simulink model "PhantomOmniSimulink"  (R2017b)
settings: Solver=VariableStepAuto  StartTime=0.0  StopTime=10.0  RelTol=1e-3
settings Model: Creator=nomad  LastModifiedBy=nomad

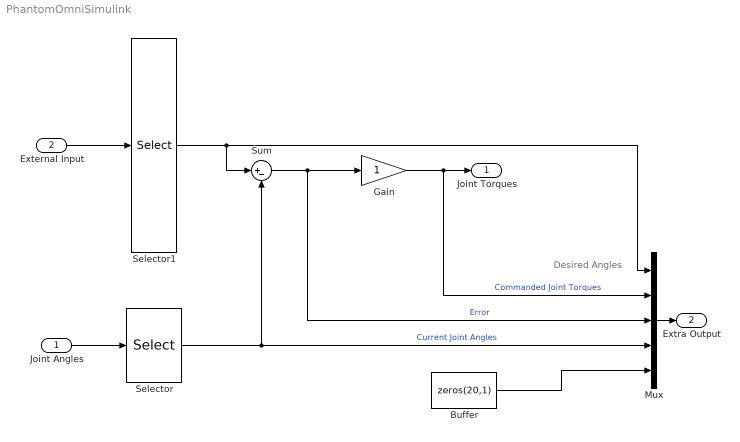
== system PhantomOmniSimulink ==
  note: Desired Angles
  Joint Angles : Inport  PortDimensions=6
  External Input : Inport  Port=2  PortDimensions=16
  Buffer : Constant  Value=zeros(20,1)
  Gain : Gain
  Mux : Mux  Inputs=5
  Selector : Selector  InputPortWidth=6  IndexOptions=Index vector (dialog)  Indices=1:3  OutputSizes=1
  Selector1 : Selector  InputPortWidth=16  IndexOptions=Index vector (dialog)  Indices=[1:3]  OutputSizes=1
  Sum : Sum  Inputs=|+-
  Joint Torques : Outport  PortDimensions=3
  Extra Output : Outport  Port=2  PortDimensions=32
  wires:
  Mux/1 -> Extra Output/1
  Joint Angles/1 -> Selector/1
  Buffer/1 -> Mux/5
  External Input/1 -> Selector1/1
  Selector/1 -> Sum/2, Mux/4  "Current Joint Angles"
  Gain/1 -> Mux/2, Joint Torques/1  "Commanded Joint Torques"
  Selector1/1 -> Sum/1, Mux/1
  Sum/1 -> Gain/1, Mux/3  "Error"
